simulink model "nonlinear_system"  (R2016a)
settings: Solver=VariableStepAuto  SolverMode=SingleTasking  StartTime=0.0  RelTol=1e-3
undefined symbols (not defined in the file or in its folder): fx, fy, izz, m, m11, m22, m26, m66, mz
settings Model: Creator=diogo  LastModifiedBy=Windows
settings DataIOCC: ReturnWorkspaceOutputs=on
settings DebuggingCC: SFUnexpectedBacktrackingDiag=error  SFNoUnconditionalDefaultTransitionDiag=error
settings SFSimCC: SimUseLocalCustomCode=on
settings RTWCC: RTWUseLocalCustomCode=on
settings GRTTargetCC: TargetLangStandard=C99 (ISO)  GeneratePreprocessorConditionals=Use local settings
settings ConfigComp: CovMetricSettings=dwe  CovHtmlReporting=off  CovSaveCumulativeToWorkspaceVar=off  CovSaveSingleToWorkspaceVar=off  CovExternalEMLEnable=on

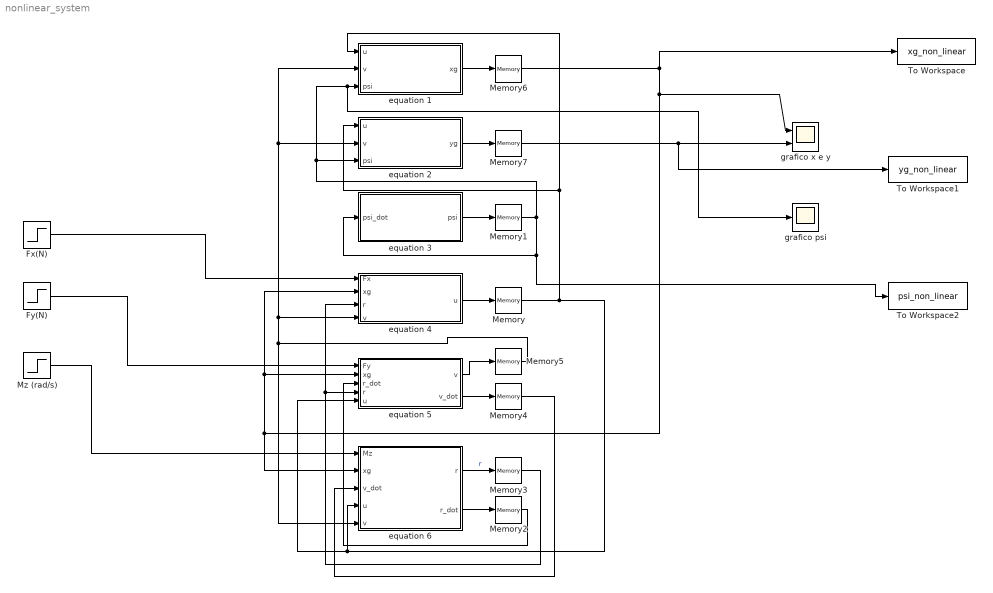
== system nonlinear_system ==
  Fx(N) : Step  Time=0  After=fx  SampleTime=0
  Fy(N) : Step  Time=0  After=fy  SampleTime=0
  Memory{,1..7} (8 alike) : Memory
  Mz (rad/s) : Step  After=mz  SampleTime=0
  To Workspace : ToWorkspace  VariableName=xg_non_linear  SaveFormat=Timeseries  SampleTime=-1
  To Workspace1 : ToWorkspace  VariableName=yg_non_linear  SaveFormat=Timeseries  SampleTime=-1
  To Workspace2 : ToWorkspace  VariableName=psi_non_linear  SaveFormat=Timeseries  SampleTime=-1
  equation 1 : Subsystem
  "equation 2 " : Subsystem
  equation 3 : Subsystem
  equation 4 : Subsystem
  equation 5 : Subsystem
  equation 6 : Subsystem
  grafico psi : Scope
  grafico x e y : Scope  NumInputPorts=2
  wires:
  Fx(N)/1 -> equation 4/1(Fx)
  Fy(N)/1 -> equation 5/1(Fy)
  Mz (rad/s)/1 -> equation 6/1(Mz)
  equation 4/1(u) -> Memory/1
  Memory/1 -> equation 1/1(u), "equation 2 "/1(u), equation 5/5(u), equation 6/4(u)
  equation 3/1(psi) -> Memory1/1
  Memory1/1 -> grafico psi/1, equation 1/3(psi), "equation 2 "/3(psi), equation 3/1(psi_dot), To Workspace2/1
  equation 6/2(r_dot) -> Memory2/1
  Memory2/1 -> equation 5/3(r_dot)
  equation 6/1(r) -> Memory3/1  "r"
  Memory3/1 -> equation 4/3(r), equation 5/4(r)
  equation 5/2(v_dot) -> Memory4/1
  Memory4/1 -> equation 6/3(v_dot)
  equation 5/1(v) -> Memory5/1
  Memory5/1 -> "equation 2 "/2(v), equation 1/2(v), equation 4/4(v), equation 6/5(v)
  Memory6/1 -> equation 4/2(xg), equation 5/2(xg), equation 6/2(xg), grafico x e y/1, To Workspace/1
  equation 1/1(xg) -> Memory6/1
  "equation 2 "/1(yg) -> Memory7/1
  Memory7/1 -> To Workspace1/1, grafico x e y/2

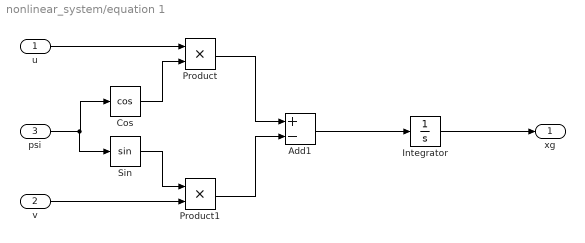
== system nonlinear_system/equation 1 ==
  u : Inport
  v : Inport  Port=2
  psi : Inport  Port=3
  Add1 : Sum  Inputs=+-
  Cos : Trigonometry  Operator=cos
  Integrator : Integrator
  Product : Product
  Product1 : Product
  Sin : Trigonometry
  xg : Outport
  wires:
  u/1 -> Product/1
  Integrator/1 -> xg/1
  psi/1 -> Sin/1, Cos/1
  Cos/1 -> Product/2
  Sin/1 -> Product1/1
  v/1 -> Product1/2
  Product/1 -> Add1/1
  Product1/1 -> Add1/2
  Add1/1 -> Integrator/1

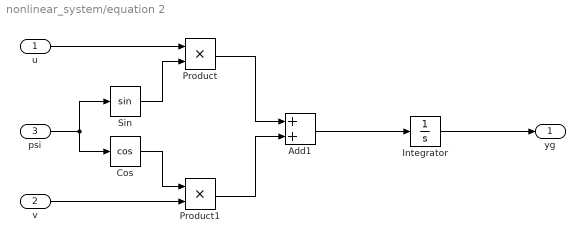
== system nonlinear_system/equation 2  ==
  u : Inport
  v : Inport  Port=2
  psi : Inport  Port=3
  Add1 : Sum
  Cos : Trigonometry  Operator=cos
  Integrator : Integrator
  Product : Product
  Product1 : Product
  Sin : Trigonometry
  yg : Outport
  wires:
  Add1/1 -> Integrator/1
  Product1/1 -> Add1/2
  Product/1 -> Add1/1
  v/1 -> Product1/2
  Sin/1 -> Product/2
  Cos/1 -> Product1/1
  psi/1 -> Sin/1, Cos/1
  Integrator/1 -> yg/1
  u/1 -> Product/1

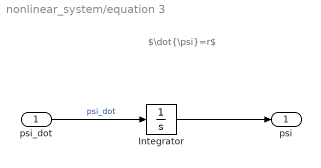
== system nonlinear_system/equation 3 ==
  note: $\dot{\psi}=r$
  psi_dot : Inport
  Integrator : Integrator
  psi : Outport
  wires:
  psi_dot/1 -> Integrator/1  "psi_dot"
  Integrator/1 -> psi/1

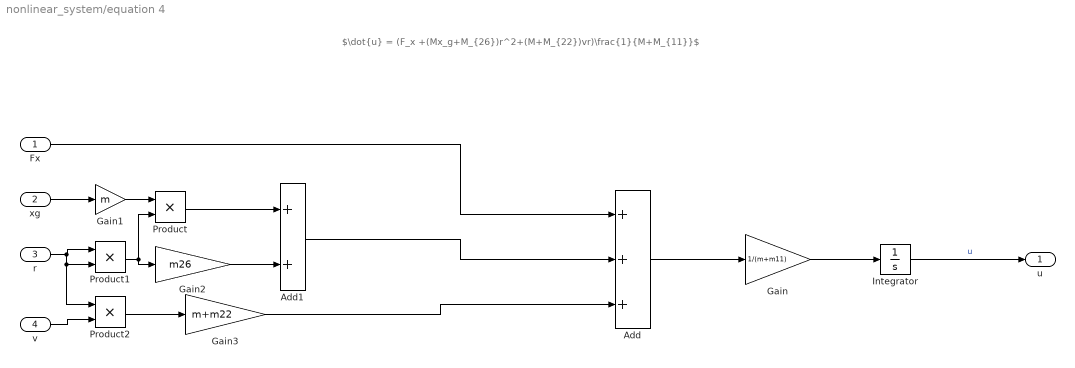
== system nonlinear_system/equation 4 ==
  note: $\dot{u} = (F_x +(Mx_g+M_{26})r^2+(M+M_{22})vr)\frac{1}{M+M_{11}}$
  Fx : Inport
  xg : Inport  Port=2
  r : Inport  Port=3
  v : Inport  Port=4
  Add : Sum  Inputs=+++
  Add1 : Sum
  Gain : Gain  Gain=1/(m+m11)
  Gain1 : Gain  Gain=m
  Gain2 : Gain  Gain=m26
  Gain3 : Gain  Gain=m+m22
  Integrator : Integrator
  Product : Product
  Product1 : Product
  Product2 : Product
  u : Outport
  wires:
  Integrator/1 -> u/1  "u"
  Gain/1 -> Integrator/1
  Add/1 -> Gain/1
  xg/1 -> Gain1/1
  Gain1/1 -> Product/1
  r/1 -> Product2/1, Product1/2, Product1/1
  Product1/1 -> Product/2, Gain2/1
  Product/1 -> Add1/1
  Gain2/1 -> Add1/2
  Add1/1 -> Add/2
  Fx/1 -> Add/1
  v/1 -> Product2/2
  Product2/1 -> Gain3/1
  Gain3/1 -> Add/3

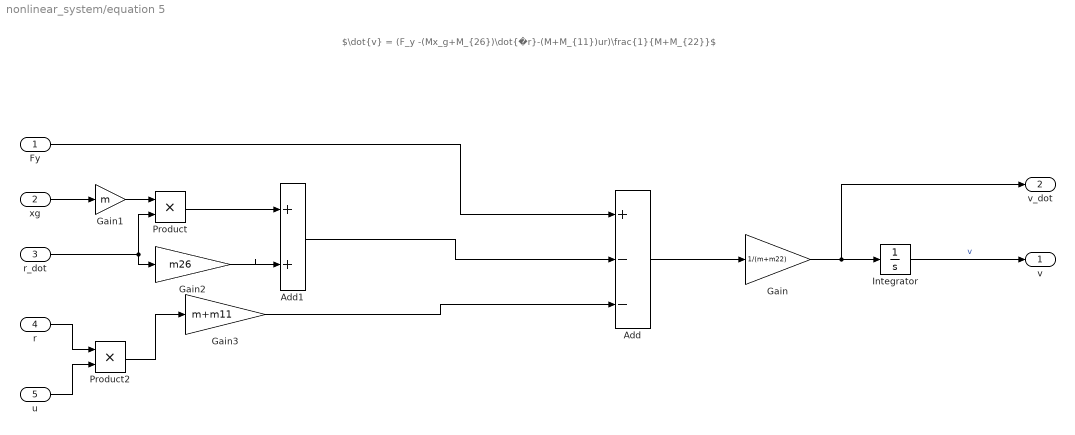
== system nonlinear_system/equation 5 ==
  note: $\dot{v} = (F_y -(Mx_g+M_{26})\dot{�r}-(M+M_{11})ur)\frac{1}{M+M_{22}}$
  Fy : Inport
  xg : Inport  Port=2
  r_dot : Inport  Port=3
  r : Inport  Port=4
  u : Inport  Port=5
  Add : Sum  Inputs=+--
  Add1 : Sum
  Gain : Gain  Gain=1/(m+m22)
  Gain1 : Gain  Gain=m
  Gain2 : Gain  Gain=m26
  Gain3 : Gain  Gain=m+m11
  Integrator : Integrator
  Product : Product
  Product2 : Product
  v : Outport
  v_dot : Outport  Port=2
  wires:
  Gain3/1 -> Add/3
  Product2/1 -> Gain3/1
  r/1 -> Product2/1
  Fy/1 -> Add/1
  Add1/1 -> Add/2
  Gain2/1 -> Add1/2
  Product/1 -> Add1/1
  r_dot/1 -> Gain2/1, Product/2
  Gain1/1 -> Product/1
  xg/1 -> Gain1/1
  Add/1 -> Gain/1
  Gain/1 -> v_dot/1, Integrator/1
  Integrator/1 -> v/1  "v"
  u/1 -> Product2/2

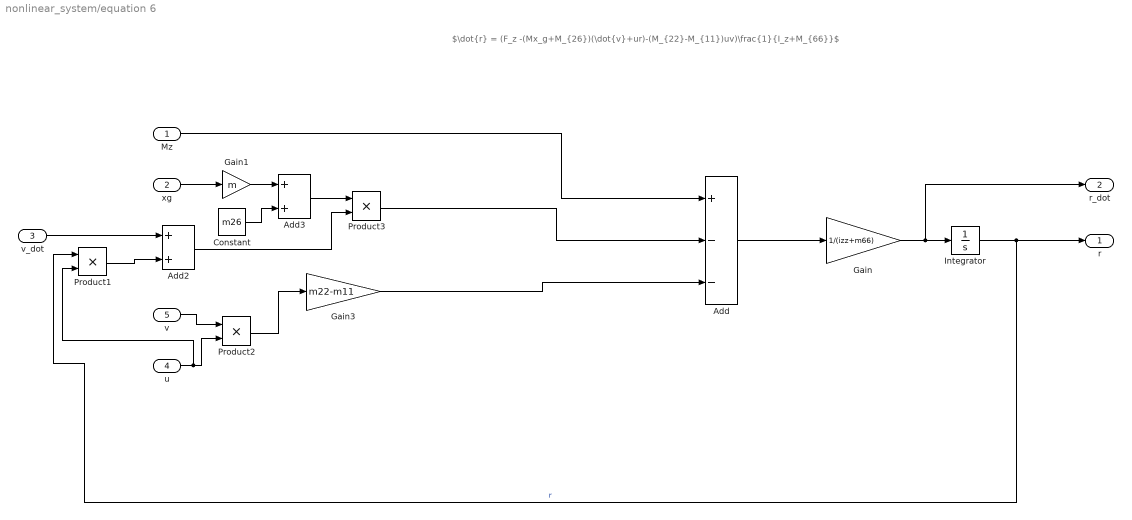
== system nonlinear_system/equation 6 ==
  note: $\dot{r} = (F_z -(Mx_g+M_{26})(\dot{v}+ur)-(M_{22}-M_{11})uv)\frac{1}{I_z+M_{66}}$
  Mz : Inport
  xg : Inport  Port=2
  v_dot : Inport  Port=3
  u : Inport  Port=4
  v : Inport  Port=5
  Add : Sum  Inputs=+--
  Add2 : Sum
  Add3 : Sum
  Constant : Constant  Value=m26
  Gain : Gain  Gain=1/(izz+m66)
  Gain1 : Gain  Gain=m
  Gain3 : Gain  Gain=m22-m11
  Integrator : Integrator
  Product1 : Product
  Product2 : Product
  Product3 : Product
  r : Outport
  r_dot : Outport  Port=2
  wires:
  u/1 -> Product1/2, Product2/2
  Integrator/1 -> Product1/1, r/1  "r"
  Gain/1 -> r_dot/1, Integrator/1
  Add/1 -> Gain/1
  xg/1 -> Gain1/1
  Gain1/1 -> Add3/1
  Product3/1 -> Add/2
  Mz/1 -> Add/1
  Product2/1 -> Gain3/1
  Gain3/1 -> Add/3
  Constant/1 -> Add3/2
  v_dot/1 -> Add2/1
  Product1/1 -> Add2/2
  Add3/1 -> Product3/1
  Add2/1 -> Product3/2
  v/1 -> Product2/1
